simulink model "lab4_dcm"  (R2021b)
settings: Solver=VariableStepAuto  StartTime=0.0  StopTime=10.0  RelTol=1e-3
values from neighbouring files (symbols this model uses):
  A0 = eye(3)    [lab4_task1and2.m]
  J = [Ixx 0 0; 0 Iyy 0; 0 0 Izz]    [lab4_task1and2.m]    (also in lab4_task3.m)
  Jinv = inv(J)    [lab4_task1and2.m]    (also in lab4_task3.m)
  w0 = [0.45 0.52 0.55]'    [lab4_task1and2.m]    (also in lab4_task3.m)
libraries: matrix_library x1
settings Model: Creator=samuz  LastModifiedBy=samuz

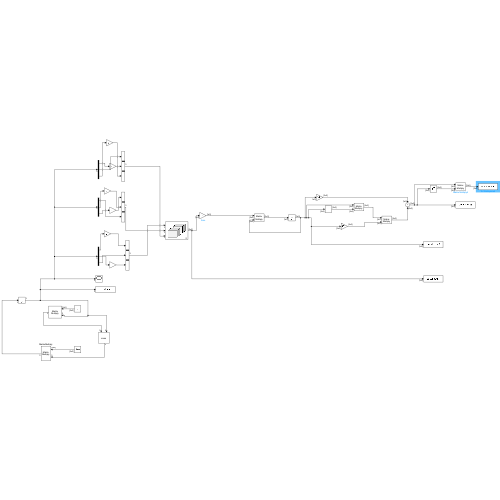
[thumbnail: Simulink's stored preview of the top-level diagram]
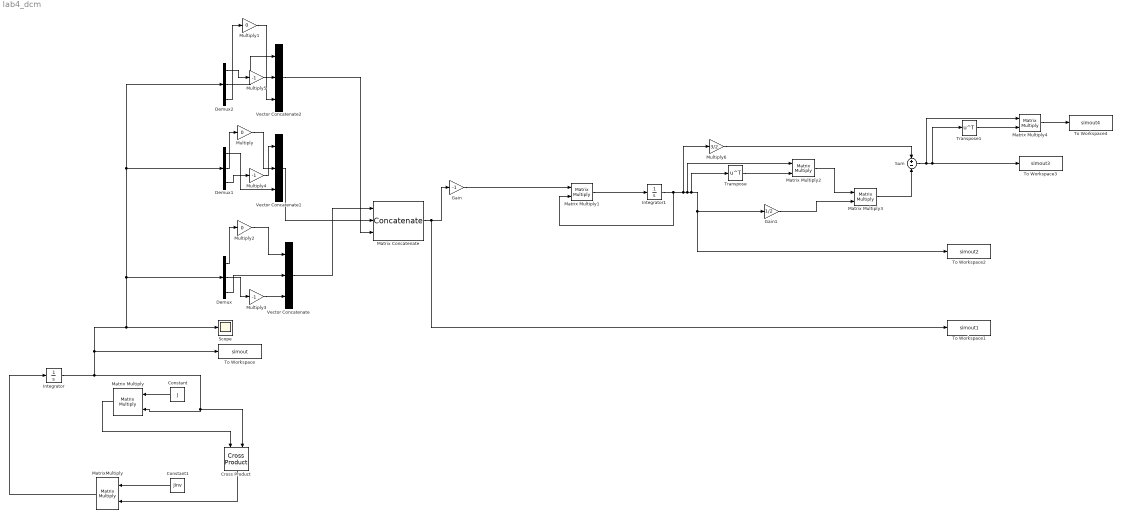
== system lab4_dcm ==
  Constant : Constant  Value=J
  Constant1 : Constant  Value=Jinv
  Cross Product : matrix_library/Cross Product
      settings: SourceProductBaseCode=SL
  Demux : Demux  Outputs=3
  Demux1 : Demux  Outputs=3
  Demux2 : Demux  Outputs=3
  Gain : Gain  Gain=-1
  Gain1 : Gain  Gain=1/2
  Integrator : Integrator  InitialCondition=w0
  Integrator1 : Integrator  InitialCondition=A0
  Matrix Concatenate : Concatenate  NumInputs=3  Mode=Multidimensional array  ConcatenateDimension=2
  Matrix Multiply{,1..4} (5 alike) : Product  Multiplication=Matrix(*)
  MatrixMultiply : Product  Multiplication=Matrix(*)
  Multiply : Gain  Gain=0
  Multiply1 : Gain  Gain=0
  Multiply2 : Gain  Gain=0
  Multiply3 : Gain  Gain=-1
  Multiply4 : Gain  Gain=-1
  Multiply5 : Gain  Gain=-1
  Multiply6 : Gain  Gain=3/2
  Scope : Scope
  Sum : Sum  Inputs=+-
  To Workspace : ToWorkspace  VariableName=simout  SampleTime=-1
  To Workspace1 : ToWorkspace  VariableName=simout1  SampleTime=-1
  To Workspace2 : ToWorkspace  VariableName=simout2  SampleTime=-1
  To Workspace3 : ToWorkspace  VariableName=simout3  SampleTime=-1
  To Workspace4 : ToWorkspace  VariableName=simout4  SampleTime=-1
  Transpose : Math  Operator=transpose  SaturateOnIntegerOverflow=on
  Transpose1 : Math  Operator=transpose  SaturateOnIntegerOverflow=on
  Vector Concatenate : Concatenate  NumInputs=3
  Vector Concatenate1 : Concatenate  NumInputs=3
  Vector Concatenate2 : Concatenate  NumInputs=3
  wires:
  Constant/1 -> Matrix Multiply/1
  MatrixMultiply/1 -> Integrator/1
  Constant1/1 -> MatrixMultiply/1
  Cross Product/1 -> MatrixMultiply/2
  Matrix Multiply/1 -> Cross Product/1
  Demux/2 -> Multiply3/1
  Integrator/1 -> To Workspace/1, Demux2/1, Demux1/1, Demux/1, Scope/1, Cross Product/2, Matrix Multiply/2
  Vector Concatenate1/1 -> Matrix Concatenate/2
  Vector Concatenate/1 -> Matrix Concatenate/1
  Demux2/2 -> Vector Concatenate2/1
  Demux2/1 -> Multiply5/1
  Demux1/2 -> Multiply/1
  Multiply/1 -> Vector Concatenate1/2
  Demux2/3 -> Multiply1/1
  Multiply1/1 -> Vector Concatenate2/3
  Demux/1 -> Multiply2/1
  Multiply2/1 -> Vector Concatenate/1
  Vector Concatenate2/1 -> Matrix Concatenate/3
  Matrix Concatenate/1 -> To Workspace1/1, Gain/1
  Demux/3 -> Vector Concatenate/2
  Multiply3/1 -> Vector Concatenate/3
  Multiply5/1 -> Vector Concatenate2/2
  Demux1/1 -> Vector Concatenate1/3
  Demux1/3 -> Multiply4/1
  Multiply4/1 -> Vector Concatenate1/1
  Gain/1 -> Matrix Multiply1/1
  Matrix Multiply1/1 -> Integrator1/1
  Integrator1/1 -> Matrix Multiply1/2, Multiply6/1, Matrix Multiply2/1, Transpose/1, Gain1/1, To Workspace2/1
  Transpose/1 -> Matrix Multiply2/2
  Matrix Multiply2/1 -> Matrix Multiply3/1
  Gain1/1 -> Matrix Multiply3/2
  Sum/1 -> Matrix Multiply4/1, Transpose1/1, To Workspace3/1
  Matrix Multiply3/1 -> Sum/2
  Multiply6/1 -> Sum/1
  Transpose1/1 -> Matrix Multiply4/2
  Matrix Multiply4/1 -> To Workspace4/1
